simulink model "agrivoltaics_v1"  (R2025b)
settings: Solver=FixedStepDiscrete  StartTime=0.0  StopTime=0  FixedStep=1  RelTol=1e-3
InitFcn:
  | agrivoltaics_variable_definition
values from neighbouring files (symbols this model uses):
  agriVar = agriVarArray2Struct(custom_var)    [agrivoltaic_wrapper.m]
undefined symbols (not defined in the file or in its folder): agriParams
libraries: crop_cost x1, crop_performance_module x1, environmental_module x1, pv_cost x1, pv_performance_module x1, value x1
settings Model: DataDictionary=agrivoltaics_v1_data_dict.sldd  Creator=ciepm  LastModifiedBy=charlielenk
settings DataIOCC: SignalLogging=off  DSMLogging=off  SaveTime=off

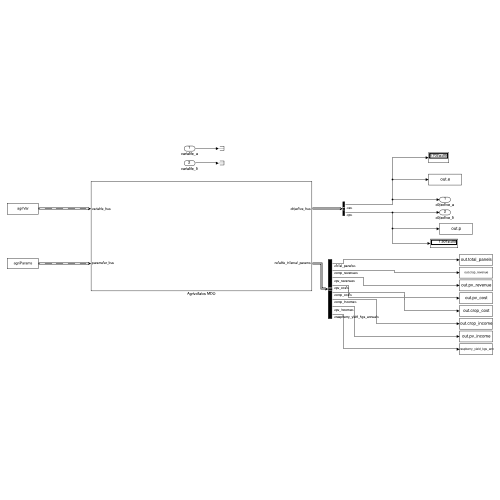
[thumbnail: Simulink's stored preview of the top-level diagram]
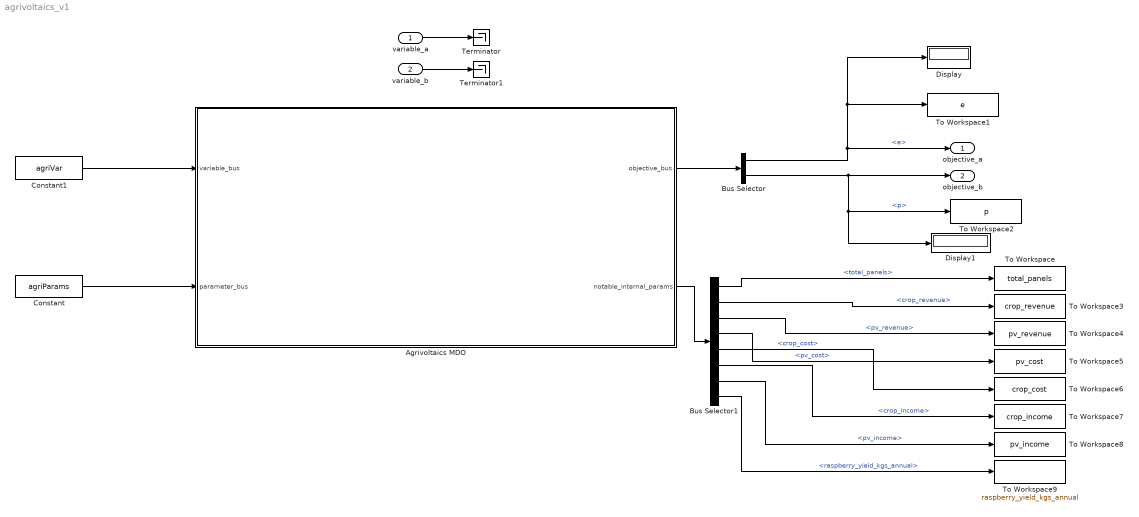
== system agrivoltaics_v1 ==
  variable_a : Inport
  variable_b : Inport  Port=2
  Agrivoltaics MDO : Subsystem
  Bus Selector : BusSelector  OutputSignals=e,p
  Bus Selector1 : BusSelector  OutputSignals=energy_per_year.total_panels,crop_revenue,pv_revenue,pv_cost,crop_cost,crop_income,pv_income,raspberry_yield_kgs_annual
  Constant : Constant  Value=agriParams  OutDataTypeStr=Bus: slBus1
  Constant1 : Constant  Value=agriVar  OutDataTypeStr=Bus: slBus2
  Display : Display
  Display1 : Display
  Terminator : Terminator
  Terminator1 : Terminator
  To Workspace : ToWorkspace  VariableName=total_panels  SaveFormat=Timeseries  SampleTime=-1
  To Workspace1 : ToWorkspace  VariableName=e  SaveFormat=Timeseries  SampleTime=-1
  To Workspace2 : ToWorkspace  VariableName=p  SaveFormat=Timeseries  SampleTime=-1
  To Workspace3 : ToWorkspace  VariableName=crop_revenue  SaveFormat=Timeseries  SampleTime=-1
  To Workspace4 : ToWorkspace  VariableName=pv_revenue  SaveFormat=Timeseries  SampleTime=-1
  To Workspace5 : ToWorkspace  VariableName=pv_cost  SaveFormat=Timeseries  SampleTime=-1
  To Workspace6 : ToWorkspace  VariableName=crop_cost  SaveFormat=Timeseries  SampleTime=-1
  To Workspace7 : ToWorkspace  VariableName=crop_income  SaveFormat=Timeseries  SampleTime=-1
  To Workspace8 : ToWorkspace  VariableName=pv_income  SaveFormat=Timeseries  SampleTime=-1
  To Workspace9 : ToWorkspace  VariableName=raspberry_yield_kgs_annual  SaveFormat=Timeseries  SampleTime=-1
  objective_a : Outport
  objective_b : Outport  Port=2
  wires:
  Agrivoltaics MDO/1(objective_bus) -> Bus Selector/1
  Bus Selector/1 -> objective_a/1, To Workspace1/1, Display/1  "<e>"
  Bus Selector/2 -> objective_b/1, To Workspace2/1, Display1/1  "<p>"
  variable_a/1 -> Terminator/1
  variable_b/1 -> Terminator1/1
  Constant1/1 -> Agrivoltaics MDO/1(variable_bus)
  Agrivoltaics MDO/2(notable_internal_params) -> Bus Selector1/1
  Bus Selector1/1 -> To Workspace/1  "<total_panels>"
  Constant/1 -> Agrivoltaics MDO/2(parameter_bus)
  Bus Selector1/2 -> To Workspace3/1  "<crop_revenue>"
  Bus Selector1/3 -> To Workspace4/1  "<pv_revenue>"
  Bus Selector1/4 -> To Workspace5/1  "<pv_cost>"
  Bus Selector1/5 -> To Workspace6/1  "<crop_cost>"
  Bus Selector1/6 -> To Workspace7/1  "<crop_income>"
  Bus Selector1/7 -> To Workspace8/1  "<pv_income>"
  Bus Selector1/8 -> To Workspace9/1  "<raspberry_yield_kgs_annual>"

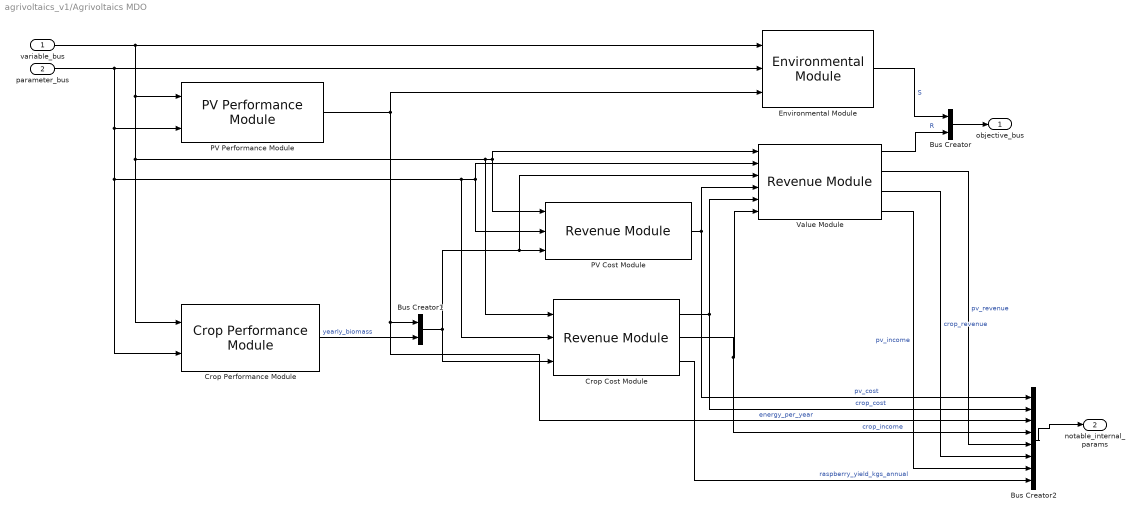
== system agrivoltaics_v1/Agrivoltaics MDO ==
  variable_bus : Inport
  parameter_bus : Inport  Port=2
  Bus Creator : BusCreator  Inputs=2  OutDataTypeStr=Bus: objective_bus
      settings: InheritFromInputs=off
  Bus Creator1 : BusCreator  Inputs=2
  Bus Creator2 : BusCreator  Inputs=8
  Crop Cost Module : crop_cost/Revenue Module  SystemSampleTime=-1  VariantActivationTime=update diagram  EmptyChoice=off  PassThrough=off  PassThroughVariantControl=(default)  EmptyChoiceVariantControl=(default)  AllowFlexibleInterface=on  Latency=0  AutoFrameSizeCalculation=off
  Crop Performance Module : crop_performance_module/Crop Performance Module  SystemSampleTime=-1  VariantActivationTime=update diagram  EmptyChoice=off  PassThrough=off  PassThroughVariantControl=(default)  EmptyChoiceVariantControl=(default)  AllowFlexibleInterface=on  Latency=0  AutoFrameSizeCalculation=off
  Environmental Module : environmental_module/Environmental Module  SystemSampleTime=-1  VariantActivationTime=update diagram  EmptyChoice=off  PassThrough=off  PassThroughVariantControl=(default)  EmptyChoiceVariantControl=(default)  AllowFlexibleInterface=on  Latency=0  AutoFrameSizeCalculation=off
  PV Cost Module : pv_cost/Revenue Module  SystemSampleTime=-1  VariantActivationTime=update diagram  EmptyChoice=off  PassThrough=off  PassThroughVariantControl=(default)  EmptyChoiceVariantControl=(default)  AllowFlexibleInterface=on  Latency=0  AutoFrameSizeCalculation=off
  PV Performance Module : pv_performance_module/PV Performance Module  SystemSampleTime=-1  VariantActivationTime=update diagram  EmptyChoice=off  PassThrough=off  PassThroughVariantControl=(default)  EmptyChoiceVariantControl=(default)  AllowFlexibleInterface=on  Latency=0  AutoFrameSizeCalculation=off
  Value Module : value/Revenue Module  SystemSampleTime=-1  VariantActivationTime=update diagram  EmptyChoice=off  PassThrough=off  PassThroughVariantControl=(default)  EmptyChoiceVariantControl=(default)  AllowFlexibleInterface=on  Latency=0  AutoFrameSizeCalculation=off
  objective_bus : Outport
  notable_internal_params : Outport  Port=2
  wires:
  variable_bus/1 -> Crop Performance Module/1, Crop Cost Module/1, PV Cost Module/1, Value Module/1, PV Performance Module/1, Environmental Module/1
  parameter_bus/1 -> Crop Performance Module/2, Crop Cost Module/2, Value Module/2, PV Cost Module/2, PV Performance Module/2, Environmental Module/2
  Crop Performance Module/1 -> Bus Creator1/2  "yearly_biomass"
  Bus Creator/1 -> objective_bus/1
  Environmental Module/1 -> Bus Creator/1  "S"
  Value Module/1 -> Bus Creator/2  "R"
  PV Performance Module/1 -> Bus Creator2/3, Bus Creator1/1, Environmental Module/3  "energy_per_year"
  Bus Creator1/1 -> Value Module/3, PV Cost Module/3, Crop Cost Module/3
  Bus Creator2/1 -> notable_internal_params/1
  PV Cost Module/1 -> Bus Creator2/1, Value Module/4  "pv_cost"
  Crop Cost Module/1 -> Bus Creator2/2, Value Module/5  "crop_cost"
  Crop Cost Module/2 -> Bus Creator2/4, Value Module/6  "crop_income"
  Value Module/2 -> Bus Creator2/5  "pv_revenue"
  Value Module/3 -> Bus Creator2/6  "crop_revenue"
  Value Module/4 -> Bus Creator2/7  "pv_income"
  Crop Cost Module/3 -> Bus Creator2/8  "raspberry_yield_kgs_annual"
